simulink library "unifier_obm"  (R2023a)
settings: Solver=VariableStepAuto  StartTime=0.0  StopTime=10.0  RelTol=1e-3
undefined symbols (not defined in the file): b, c, dp_DEP, dp_FUSE_FIN, dp_HTU, dp_VTAIL, dp_VTAIL_INDUCED, dp_WING_root, dp_WING_tip, I, m, S, vtail_nodes, wing_nodes, xyz_cg, xyz_DEP
libraries: sharedutil x7, aerolibtransform2 x4, sharedtransform x2, matrix_library x1, shared6dofsys x1, shared6dof x1, simulink x1
(part 2 of 2)

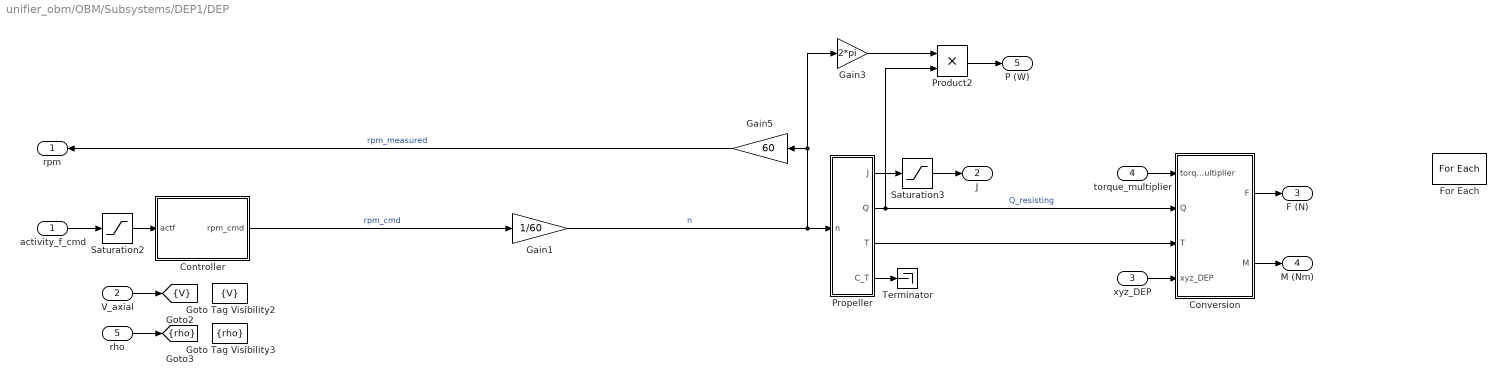
== system unifier_obm/OBM/Subsystems/DEP1/DEP ==
  activity_f_cmd : Inport  Partition=on  PartitionDimension=1  PartitionWidth=1  PartitionOffset=0
  V_axial : Inport  Port=2  Partition=on  PartitionDimension=1  PartitionWidth=1  PartitionOffset=0
  xyz_DEP : Inport  Port=3  Partition=on  PartitionDimension=2  PartitionWidth=1  PartitionOffset=0
  torque_multiplier : Inport  Port=4  Partition=on  PartitionDimension=1  PartitionWidth=1  PartitionOffset=0
  rho : Inport  Port=5
  Controller : Subsystem
  Conversion : Subsystem
  For Each : ForEach  DisableCoverage=on  SpecifiedNumIters=12
  Gain1 : Gain  Gain=1/60
  Gain3 : Gain  Gain=2*pi
  Gain5 : Gain  Gain=60
  Goto Tag Visibility2 : GotoTagVisibility  GotoTag=V
  Goto Tag Visibility3 : GotoTagVisibility  GotoTag=rho
  Product2 : Product
  Propeller : Subsystem
  Saturation2 : Saturate  UpperLimit=1  LowerLimit=0
  Saturation3 : Saturate  UpperLimit=5  LowerLimit=0.2
  Terminator : Terminator
  rpm : Outport  ConcatenationDimension=1
  J : Outport  Port=2  ConcatenationDimension=1
  F (N) : Outport  Port=3  ConcatenationDimension=2
  M (Nm) : Outport  Port=4  ConcatenationDimension=2
  P (W) : Outport  Port=5  ConcatenationDimension=1
  tag scope: V=scoped, rho=scoped
  wires:
  Conversion/1(F) -> F (N)/1
  Conversion/2(M) -> M (Nm)/1
  Saturation3/1 -> J/1
  Propeller/4(C_T) -> Terminator/1
  activity_f_cmd/1 -> Saturation2/1
  Propeller/1(J) -> Saturation3/1
  Gain3/1 -> Product2/1
  xyz_DEP/1 -> Conversion/4(xyz_DEP)
  Gain1/1 -> Gain3/1, Gain5/1, Propeller/1(n)  "n"
  V_axial/1 -> [V]
  Product2/1 -> P (W)/1
  torque_multiplier/1 -> Conversion/1(torque_multiplier)
  Gain5/1 -> rpm/1  "rpm_measured"
  Propeller/3(T) -> Conversion/3(T)
  rho/1 -> [rho]
  Propeller/2(Q) -> Product2/2, Conversion/2(Q)  "Q_resisting"
  Saturation2/1 -> Controller/1(actf)
  Controller/1(rpm_cmd) -> Gain1/1  "rpm_cmd"

== system unifier_obm/OBM/Subsystems/HTU/PropAndMotor ==
  Vrw_mag_eas : Inport
  T_cmd (N) : Inport  Port=2
  1-D Lookup Table : Lookup_n-D  NumberOfTableDimensions=1  BreakpointsForDimension1=dp_HTU.limits.V_low_lim  IndexSearchMethod=Linear search  BeginIndexSearchUsingPreviousIndexResult=on  Table=dp_HTU.limits.T_low_lim  InternalRulePriority=Speed  RndMeth=Simplest
  1-D Lookup Table1 : Lookup_n-D  NumberOfTableDimensions=1  BreakpointsForDimension1=dp_HTU.limits.V_up_lim  IndexSearchMethod=Linear search  BeginIndexSearchUsingPreviousIndexResult=on  Table=dp_HTU.limits.T_up_lim  InternalRulePriority=Speed  RndMeth=Simplest
  P lookup : Lookup_n-D  BreakpointsForDimension1=dp_HTU.V_vec  BreakpointsForDimension2=dp_HTU.T_vec  IndexSearchMethod=Linear search  BeginIndexSearchUsingPreviousIndexResult=on  Table=dp_HTU.P_grid  InternalRulePriority=Speed  RndMeth=Simplest
      settings: InputPortMap=u0,u1
  Saturation Dynamic : simulink/Discontinuities/Saturation Dynamic  OutMin=[]  OutMax=[]  OutDataTypeStr=Inherit: Same as second input  OutDataType=fixdt(1, 16)  OutScaling=2^-10  DoSatur=off
  P (kW) : Outport
  T (N) : Outport  Port=2
  wires:
  Vrw_mag_eas/1 -> P lookup/1, 1-D Lookup Table/1, 1-D Lookup Table1/1
  P lookup/1 -> P (kW)/1
  1-D Lookup Table1/1 -> Saturation Dynamic/1
  1-D Lookup Table/1 -> Saturation Dynamic/3
  T_cmd (N)/1 -> Saturation Dynamic/2
  Saturation Dynamic/1 -> T (N)/1, P lookup/2

== system unifier_obm/OBM/Aero/FinFuselageForces/Subsystem1/Subsystem ==
  beta : Inport
  alpha : Inport  Port=2
  Prelookup : PreLookup  BreakpointsData=dp_FUSE_FIN.beta  IndexSearchMethod=Linear search  BeginIndexSearchUsingPreviousIndexResult=on  ExtrapMethod=Linear
  Prelookup1 : PreLookup  BreakpointsData=dp_FUSE_FIN.aoa  IndexSearchMethod=Linear search  BeginIndexSearchUsingPreviousIndexResult=on  ExtrapMethod=Linear
  Out1 : Outport
  Out2 : Outport  Port=2
  Out3 : Outport  Port=3
  Out4 : Outport  Port=4
  wires:
  Prelookup/1 -> Out1/1
  alpha/1 -> Prelookup1/1
  beta/1 -> Prelookup/1
  Prelookup1/1 -> Out3/1
  Prelookup1/2 -> Out4/1
  Prelookup/2 -> Out2/1

== system unifier_obm/OBM/Aero/VtailForces/Subsystem/CrossProduct1 ==
  r : Inport  Partition=on  PartitionDimension=2  PartitionWidth=1  PartitionOffset=0
  F : Inport  Port=2  Partition=on  PartitionDimension=2  PartitionWidth=1  PartitionOffset=0
  3x3 Cross Product : sharedutil/3x3 Cross Product  aMode=aMode
  CG : Constant  Value=xyz_cg
  Cast : DataTypeConversion  OutDataTypeStr=single  SaturateOnIntegerOverflow=off  RndMeth=Floor
  For Each : ForEach  DisableCoverage=on  SpecifiedNumIters=16
  Minus : Sum  Inputs=+-
  M : Outport  ConcatenationDimension=2
  wires:
  F/1 -> 3x3 Cross Product/2
  r/1 -> Minus/1
  3x3 Cross Product/1 -> M/1
  CG/1 -> Cast/1
  Minus/1 -> 3x3 Cross Product/1
  Cast/1 -> Minus/2

== system unifier_obm/OBM/Aero/VtailForces/VtailForces/WingRootPreLookup ==
  rude_defl_nodes : Inport
  alpha_nodes : Inport  Port=2
  beta_nodes : Inport  Port=3
  Constant8 : Constant  Value=0:15
  Prelookup : PreLookup  BreakpointsData=dp_VTAIL.rude_defl  IndexSearchMethod=Linear search  BeginIndexSearchUsingPreviousIndexResult=on  ExtrapMethod=Linear
  Prelookup1 : PreLookup  BreakpointsData=dp_VTAIL.alphas  IndexSearchMethod=Linear search  BeginIndexSearchUsingPreviousIndexResult=on  ExtrapMethod=Linear
  Prelookup2 : PreLookup  BreakpointsData=dp_VTAIL.betas  IndexSearchMethod=Linear search  BeginIndexSearchUsingPreviousIndexResult=on  ExtrapMethod=Linear
  Out1 : Outport
  Out2 : Outport  Port=2
  Out3 : Outport  Port=3
  Out4 : Outport  Port=4
  Out6 : Outport  Port=5
  Out7 : Outport  Port=6
  Out5 : Outport  Port=7
  wires:
  Prelookup/1 -> Out1/1
  Constant8/1 -> Out5/1
  Prelookup1/2 -> Out4/1
  Prelookup/2 -> Out2/1
  alpha_nodes/1 -> Prelookup1/1
  Prelookup1/1 -> Out3/1
  rude_defl_nodes/1 -> Prelookup/1
  beta_nodes/1 -> Prelookup2/1
  Prelookup2/1 -> Out6/1
  Prelookup2/2 -> Out7/1

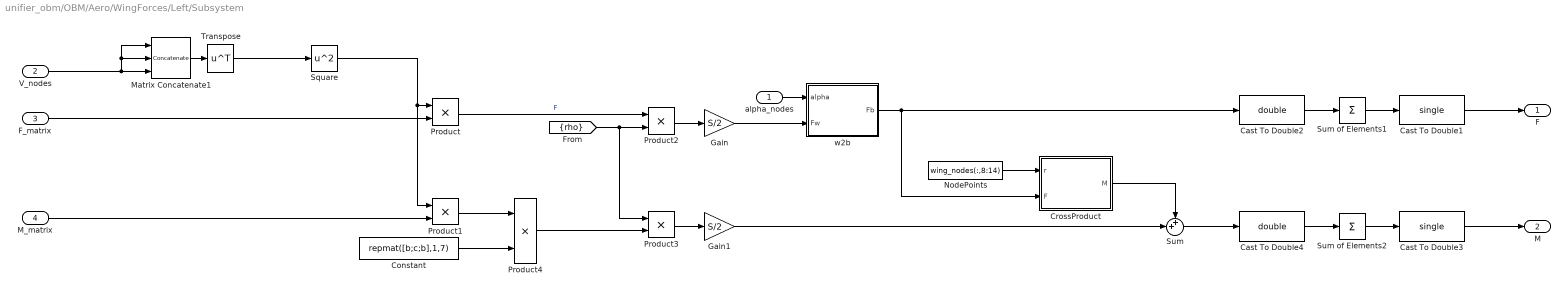
== system unifier_obm/OBM/Aero/WingForces/Left/Subsystem ==
  alpha_nodes : Inport
  V_nodes : Inport  Port=2
  F_matrix : Inport  Port=3
  M_matrix : Inport  Port=4
  Cast To Double1 : DataTypeConversion  OutDataTypeStr=single  SaturateOnIntegerOverflow=off  RndMeth=Floor
  Cast To Double2 : DataTypeConversion  OutDataTypeStr=double  SaturateOnIntegerOverflow=off  RndMeth=Floor
  Cast To Double3 : DataTypeConversion  OutDataTypeStr=single  SaturateOnIntegerOverflow=off  RndMeth=Floor
  Cast To Double4 : DataTypeConversion  OutDataTypeStr=double  SaturateOnIntegerOverflow=off  RndMeth=Floor
  Constant : Constant  Value=repmat([b;c;b],1,7)
  CrossProduct : Subsystem  TreatAsAtomicUnit=on
  Gain : Gain  Gain=S/2
  Gain1 : Gain  Gain=S/2
  Matrix Concatenate1 : Concatenate  NumInputs=3  Mode=Multidimensional array  ConcatenateDimension=2
  NodePoints : Constant  Value=wing_nodes(:,8:14)
  Product{,1..4} (5 alike) : Product
  Square : Math  Operator=square
  Sum : Sum  Inputs=++|
  Sum of Elements1 : Sum  Inputs=+  CollapseMode=Specified dimension  CollapseDim=2
  Sum of Elements2 : Sum  Inputs=+  CollapseMode=Specified dimension  CollapseDim=2
  Transpose : Math  Operator=transpose
  w2b : Subsystem  TreatAsAtomicUnit=on
  F : Outport
  M : Outport  Port=2
  wires:
  Product2/1 -> Gain/1
  F_matrix/1 -> Product/2
  [rho] -> Product3/1, Product2/2
  Product3/1 -> Gain1/1
  Constant/1 -> Product4/2
  Product4/1 -> Product3/2
  M_matrix/1 -> Product1/2
  Product1/1 -> Product4/1
  Gain1/1 -> Sum/2
  Product/1 -> Product2/1  "F"
  V_nodes/1 -> Matrix Concatenate1/1, Matrix Concatenate1/2, Matrix Concatenate1/3
  Transpose/1 -> Square/1
  Matrix Concatenate1/1 -> Transpose/1
  Square/1 -> Product1/1, Product/1
  w2b/1(Fb) -> Cast To Double2/1, CrossProduct/2(F)
  NodePoints/1 -> CrossProduct/1(r)
  CrossProduct/1(M) -> Sum/1
  Cast To Double1/1 -> F/1
  Gain/1 -> w2b/2(Fw)
  alpha_nodes/1 -> w2b/1(alpha)
  Cast To Double2/1 -> Sum of Elements1/1
  Sum of Elements1/1 -> Cast To Double1/1
  Sum of Elements2/1 -> Cast To Double3/1
  Cast To Double4/1 -> Sum of Elements2/1
  Sum/1 -> Cast To Double4/1
  Cast To Double3/1 -> M/1

== system unifier_obm/OBM/Aero/WingForces/Left/WingRootForces ==
  flap_defl : Inport
  alpha : Inport  Port=2
  V_node : Inport  Port=3
  DEP_J : Inport  Port=4
  Interpolation Using Prelookup1 : Interpolation_n-D  NumberOfTableDimensions=5  Table=dp_WING_root.CD  ExtrapMethod=Clip  ValidIndexMayReachLast=on  NumSelectionDims=1  InternalRulePriority=Speed  TableDataTypeStr=Inherit: Inherit from 'Table data'
      settings: InputPortMap=u0,u1,u2,u3,u4,u5,u6,u7,u8
  Interpolation Using Prelookup2 : Interpolation_n-D  NumberOfTableDimensions=5  Table=dp_WING_root.CS  ExtrapMethod=Clip  ValidIndexMayReachLast=on  NumSelectionDims=1  InternalRulePriority=Speed  TableDataTypeStr=Inherit: Inherit from 'Table data'
      settings: InputPortMap=u0,u1,u2,u3,u4,u5,u6,u7,u8
  Interpolation Using Prelookup3 : Interpolation_n-D  NumberOfTableDimensions=5  Table=dp_WING_root.CL  ExtrapMethod=Clip  ValidIndexMayReachLast=on  NumSelectionDims=1  InternalRulePriority=Speed  TableDataTypeStr=Inherit: Inherit from 'Table data'
      settings: InputPortMap=u0,u1,u2,u3,u4,u5,u6,u7,u8
  Interpolation Using Prelookup4 : Interpolation_n-D  NumberOfTableDimensions=5  Table=dp_WING_root.CMx  ExtrapMethod=Clip  ValidIndexMayReachLast=on  NumSelectionDims=1  InternalRulePriority=Speed  TableDataTypeStr=Inherit: Inherit from 'Table data'
      settings: InputPortMap=u0,u1,u2,u3,u4,u5,u6,u7,u8
  Interpolation Using Prelookup5 : Interpolation_n-D  NumberOfTableDimensions=5  Table=dp_WING_root.CMy  ExtrapMethod=Clip  ValidIndexMayReachLast=on  NumSelectionDims=1  InternalRulePriority=Speed  TableDataTypeStr=Inherit: Inherit from 'Table data'
      settings: InputPortMap=u0,u1,u2,u3,u4,u5,u6,u7,u8
  Interpolation Using Prelookup6 : Interpolation_n-D  NumberOfTableDimensions=5  Table=dp_WING_root.CMz  ExtrapMethod=Clip  ValidIndexMayReachLast=on  NumSelectionDims=1  InternalRulePriority=Speed  TableDataTypeStr=Inherit: Inherit from 'Table data'
      settings: InputPortMap=u0,u1,u2,u3,u4,u5,u6,u7,u8
  WingRootPreLookup : Subsystem
  CD : Outport
  CS : Outport  Port=2
  CL : Outport  Port=3
  CMx : Outport  Port=4
  CMy : Outport  Port=5
  CMz : Outport  Port=6
  wires:
  WingRootPreLookup/9(Out5) -> Interpolation Using Prelookup6/9, Interpolation Using Prelookup5/9, Interpolation Using Prelookup4/9, Interpolation Using Prelookup3/9, Interpolation Using Prelookup2/9, Interpolation Using Prelookup1/9
  WingRootPreLookup/3(Out3) -> Interpolation Using Prelookup6/3, Interpolation Using Prelookup5/3, Interpolation Using Prelookup4/3, Interpolation Using Prelookup3/3, Interpolation Using Prelookup2/3, Interpolation Using Prelookup1/3
  WingRootPreLookup/8(Out9) -> Interpolation Using Prelookup6/8, Interpolation Using Prelookup5/8, Interpolation Using Prelookup4/8, Interpolation Using Prelookup3/8, Interpolation Using Prelookup2/8, Interpolation Using Prelookup1/8
  WingRootPreLookup/1(Out1) -> Interpolation Using Prelookup6/1, Interpolation Using Prelookup5/1, Interpolation Using Prelookup4/1, Interpolation Using Prelookup3/1, Interpolation Using Prelookup2/1, Interpolation Using Prelookup1/1
  WingRootPreLookup/7(Out8) -> Interpolation Using Prelookup1/7, Interpolation Using Prelookup5/7, Interpolation Using Prelookup6/7, Interpolation Using Prelookup4/7, Interpolation Using Prelookup3/7, Interpolation Using Prelookup2/7
  flap_defl/1 -> WingRootPreLookup/1(flap_defl)
  WingRootPreLookup/4(Out4) -> Interpolation Using Prelookup6/4, Interpolation Using Prelookup5/4, Interpolation Using Prelookup4/4, Interpolation Using Prelookup3/4, Interpolation Using Prelookup2/4, Interpolation Using Prelookup1/4
  WingRootPreLookup/5(Out6) -> Interpolation Using Prelookup1/5, Interpolation Using Prelookup6/5, Interpolation Using Prelookup5/5, Interpolation Using Prelookup4/5, Interpolation Using Prelookup3/5, Interpolation Using Prelookup2/5
  Interpolation Using Prelookup1/1 -> CD/1
  WingRootPreLookup/6(Out7) -> Interpolation Using Prelookup6/6, Interpolation Using Prelookup5/6, Interpolation Using Prelookup4/6, Interpolation Using Prelookup3/6, Interpolation Using Prelookup2/6, Interpolation Using Prelookup1/6
  WingRootPreLookup/2(Out2) -> Interpolation Using Prelookup6/2, Interpolation Using Prelookup5/2, Interpolation Using Prelookup4/2, Interpolation Using Prelookup3/2, Interpolation Using Prelookup2/2, Interpolation Using Prelookup1/2
  DEP_J/1 -> WingRootPreLookup/4(DEP_J)
  V_node/1 -> WingRootPreLookup/3(V_node)
  alpha/1 -> WingRootPreLookup/2(alpha)
  Interpolation Using Prelookup2/1 -> CS/1
  Interpolation Using Prelookup3/1 -> CL/1
  Interpolation Using Prelookup4/1 -> CMx/1
  Interpolation Using Prelookup5/1 -> CMy/1
  Interpolation Using Prelookup6/1 -> CMz/1

== system unifier_obm/OBM/Aero/WingForces/Left/WingTipForces ==
  ail_defl : Inport
  alpha : Inport  Port=2
  V_node : Inport  Port=3
  DEP_J : Inport  Port=4
  Interpolation Using Prelookup1 : Interpolation_n-D  NumberOfTableDimensions=5  Table=dp_WING_tip.CD  ExtrapMethod=Clip  ValidIndexMayReachLast=on  NumSelectionDims=1  InternalRulePriority=Speed  TableDataTypeStr=Inherit: Inherit from 'Table data'
      settings: InputPortMap=u0,u1,u2,u3,u4,u5,u6,u7,u8
  Interpolation Using Prelookup2 : Interpolation_n-D  NumberOfTableDimensions=5  Table=dp_WING_tip.CS  ExtrapMethod=Clip  ValidIndexMayReachLast=on  NumSelectionDims=1  InternalRulePriority=Speed  TableDataTypeStr=Inherit: Inherit from 'Table data'
      settings: InputPortMap=u0,u1,u2,u3,u4,u5,u6,u7,u8
  Interpolation Using Prelookup3 : Interpolation_n-D  NumberOfTableDimensions=5  Table=dp_WING_tip.CL  ExtrapMethod=Clip  ValidIndexMayReachLast=on  NumSelectionDims=1  InternalRulePriority=Speed  TableDataTypeStr=Inherit: Inherit from 'Table data'
      settings: InputPortMap=u0,u1,u2,u3,u4,u5,u6,u7,u8
  Interpolation Using Prelookup4 : Interpolation_n-D  NumberOfTableDimensions=5  Table=dp_WING_tip.CMx  ExtrapMethod=Clip  ValidIndexMayReachLast=on  NumSelectionDims=1  InternalRulePriority=Speed  TableDataTypeStr=Inherit: Inherit from 'Table data'
      settings: InputPortMap=u0,u1,u2,u3,u4,u5,u6,u7,u8
  Interpolation Using Prelookup5 : Interpolation_n-D  NumberOfTableDimensions=5  Table=dp_WING_tip.CMy  ExtrapMethod=Clip  ValidIndexMayReachLast=on  NumSelectionDims=1  InternalRulePriority=Speed  TableDataTypeStr=Inherit: Inherit from 'Table data'
      settings: InputPortMap=u0,u1,u2,u3,u4,u5,u6,u7,u8
  Interpolation Using Prelookup6 : Interpolation_n-D  NumberOfTableDimensions=5  Table=dp_WING_tip.CMz  ExtrapMethod=Clip  ValidIndexMayReachLast=on  NumSelectionDims=1  InternalRulePriority=Speed  TableDataTypeStr=Inherit: Inherit from 'Table data'
      settings: InputPortMap=u0,u1,u2,u3,u4,u5,u6,u7,u8
  WingRootPreLookup : Subsystem
  CD : Outport
  CS : Outport  Port=2
  CL : Outport  Port=3
  CMx : Outport  Port=4
  CMy : Outport  Port=5
  CMz : Outport  Port=6
  wires:
  WingRootPreLookup/9(Out5) -> Interpolation Using Prelookup6/9, Interpolation Using Prelookup5/9, Interpolation Using Prelookup4/9, Interpolation Using Prelookup3/9, Interpolation Using Prelookup2/9, Interpolation Using Prelookup1/9
  WingRootPreLookup/3(Out3) -> Interpolation Using Prelookup6/3, Interpolation Using Prelookup5/3, Interpolation Using Prelookup4/3, Interpolation Using Prelookup3/3, Interpolation Using Prelookup2/3, Interpolation Using Prelookup1/3
  WingRootPreLookup/8(Out9) -> Interpolation Using Prelookup6/8, Interpolation Using Prelookup5/8, Interpolation Using Prelookup4/8, Interpolation Using Prelookup3/8, Interpolation Using Prelookup2/8, Interpolation Using Prelookup1/8
  WingRootPreLookup/1(Out1) -> Interpolation Using Prelookup6/1, Interpolation Using Prelookup5/1, Interpolation Using Prelookup4/1, Interpolation Using Prelookup3/1, Interpolation Using Prelookup2/1, Interpolation Using Prelookup1/1
  WingRootPreLookup/7(Out8) -> Interpolation Using Prelookup5/7, Interpolation Using Prelookup6/7, Interpolation Using Prelookup4/7, Interpolation Using Prelookup3/7, Interpolation Using Prelookup2/7, Interpolation Using Prelookup1/7
  ail_defl/1 -> WingRootPreLookup/1(ail_defl)
  WingRootPreLookup/4(Out4) -> Interpolation Using Prelookup6/4, Interpolation Using Prelookup5/4, Interpolation Using Prelookup4/4, Interpolation Using Prelookup3/4, Interpolation Using Prelookup2/4, Interpolation Using Prelookup1/4
  WingRootPreLookup/5(Out6) -> Interpolation Using Prelookup1/5, Interpolation Using Prelookup6/5, Interpolation Using Prelookup5/5, Interpolation Using Prelookup4/5, Interpolation Using Prelookup3/5, Interpolation Using Prelookup2/5
  Interpolation Using Prelookup1/1 -> CD/1
  WingRootPreLookup/6(Out7) -> Interpolation Using Prelookup6/6, Interpolation Using Prelookup5/6, Interpolation Using Prelookup4/6, Interpolation Using Prelookup3/6, Interpolation Using Prelookup2/6, Interpolation Using Prelookup1/6
  WingRootPreLookup/2(Out2) -> Interpolation Using Prelookup6/2, Interpolation Using Prelookup5/2, Interpolation Using Prelookup4/2, Interpolation Using Prelookup3/2, Interpolation Using Prelookup2/2, Interpolation Using Prelookup1/2
  DEP_J/1 -> WingRootPreLookup/4(DEP_J)
  V_node/1 -> WingRootPreLookup/3(V_node)
  alpha/1 -> WingRootPreLookup/2(alpha)
  Interpolation Using Prelookup2/1 -> CS/1
  Interpolation Using Prelookup3/1 -> CL/1
  Interpolation Using Prelookup4/1 -> CMx/1
  Interpolation Using Prelookup5/1 -> CMy/1
  Interpolation Using Prelookup6/1 -> CMz/1

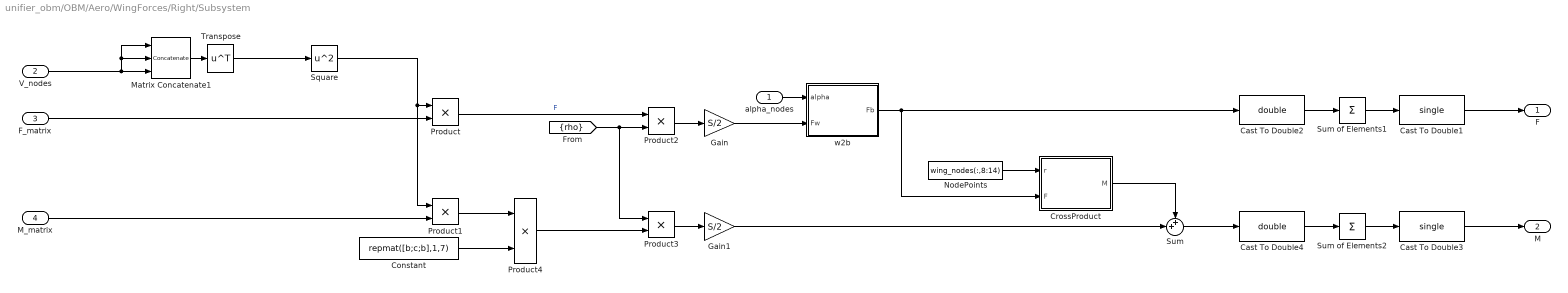
== system unifier_obm/OBM/Aero/WingForces/Right/Subsystem ==
  alpha_nodes : Inport
  V_nodes : Inport  Port=2
  F_matrix : Inport  Port=3
  M_matrix : Inport  Port=4
  Cast To Double1 : DataTypeConversion  OutDataTypeStr=single  SaturateOnIntegerOverflow=off  RndMeth=Floor
  Cast To Double2 : DataTypeConversion  OutDataTypeStr=double  SaturateOnIntegerOverflow=off  RndMeth=Floor
  Cast To Double3 : DataTypeConversion  OutDataTypeStr=single  SaturateOnIntegerOverflow=off  RndMeth=Floor
  Cast To Double4 : DataTypeConversion  OutDataTypeStr=double  SaturateOnIntegerOverflow=off  RndMeth=Floor
  Constant : Constant  Value=repmat([b;c;b],1,7)
  CrossProduct : Subsystem  TreatAsAtomicUnit=on
  Gain : Gain  Gain=S/2
  Gain1 : Gain  Gain=S/2
  Matrix Concatenate1 : Concatenate  NumInputs=3  Mode=Multidimensional array  ConcatenateDimension=2
  NodePoints : Constant  Value=wing_nodes(:,8:14)
  Product{,1..4} (5 alike) : Product
  Square : Math  Operator=square
  Sum : Sum  Inputs=++|
  Sum of Elements1 : Sum  Inputs=+  CollapseMode=Specified dimension  CollapseDim=2
  Sum of Elements2 : Sum  Inputs=+  CollapseMode=Specified dimension  CollapseDim=2
  Transpose : Math  Operator=transpose
  w2b : Subsystem  TreatAsAtomicUnit=on
  F : Outport
  M : Outport  Port=2
  wires:
  Product2/1 -> Gain/1
  F_matrix/1 -> Product/2
  [rho] -> Product3/1, Product2/2
  Product3/1 -> Gain1/1
  Constant/1 -> Product4/2
  Product4/1 -> Product3/2
  M_matrix/1 -> Product1/2
  Product1/1 -> Product4/1
  Gain1/1 -> Sum/2
  Product/1 -> Product2/1  "F"
  V_nodes/1 -> Matrix Concatenate1/1, Matrix Concatenate1/2, Matrix Concatenate1/3
  Transpose/1 -> Square/1
  Matrix Concatenate1/1 -> Transpose/1
  Square/1 -> Product1/1, Product/1
  w2b/1(Fb) -> Cast To Double2/1, CrossProduct/2(F)
  NodePoints/1 -> CrossProduct/1(r)
  CrossProduct/1(M) -> Sum/1
  Cast To Double1/1 -> F/1
  Gain/1 -> w2b/2(Fw)
  alpha_nodes/1 -> w2b/1(alpha)
  Cast To Double2/1 -> Sum of Elements1/1
  Sum of Elements1/1 -> Cast To Double1/1
  Sum of Elements2/1 -> Cast To Double3/1
  Cast To Double4/1 -> Sum of Elements2/1
  Sum/1 -> Cast To Double4/1
  Cast To Double3/1 -> M/1

== system unifier_obm/OBM/Aero/WingForces/Right/WingRootForces ==
  flap_defl : Inport
  alpha : Inport  Port=2
  V_node : Inport  Port=3
  DEP_J : Inport  Port=4
  Interpolation Using Prelookup1 : Interpolation_n-D  NumberOfTableDimensions=5  Table=dp_WING_root.CD  ExtrapMethod=Clip  ValidIndexMayReachLast=on  NumSelectionDims=1  InternalRulePriority=Speed  TableDataTypeStr=Inherit: Inherit from 'Table data'
      settings: InputPortMap=u0,u1,u2,u3,u4,u5,u6,u7,u8
  Interpolation Using Prelookup2 : Interpolation_n-D  NumberOfTableDimensions=5  Table=dp_WING_root.CS  ExtrapMethod=Clip  ValidIndexMayReachLast=on  NumSelectionDims=1  InternalRulePriority=Speed  TableDataTypeStr=Inherit: Inherit from 'Table data'
      settings: InputPortMap=u0,u1,u2,u3,u4,u5,u6,u7,u8
  Interpolation Using Prelookup3 : Interpolation_n-D  NumberOfTableDimensions=5  Table=dp_WING_root.CL  ExtrapMethod=Clip  ValidIndexMayReachLast=on  NumSelectionDims=1  InternalRulePriority=Speed  TableDataTypeStr=Inherit: Inherit from 'Table data'
      settings: InputPortMap=u0,u1,u2,u3,u4,u5,u6,u7,u8
  Interpolation Using Prelookup4 : Interpolation_n-D  NumberOfTableDimensions=5  Table=dp_WING_root.CMx  ExtrapMethod=Clip  ValidIndexMayReachLast=on  NumSelectionDims=1  InternalRulePriority=Speed  TableDataTypeStr=Inherit: Inherit from 'Table data'
      settings: InputPortMap=u0,u1,u2,u3,u4,u5,u6,u7,u8
  Interpolation Using Prelookup5 : Interpolation_n-D  NumberOfTableDimensions=5  Table=dp_WING_root.CMy  ExtrapMethod=Clip  ValidIndexMayReachLast=on  NumSelectionDims=1  InternalRulePriority=Speed  TableDataTypeStr=Inherit: Inherit from 'Table data'
      settings: InputPortMap=u0,u1,u2,u3,u4,u5,u6,u7,u8
  Interpolation Using Prelookup6 : Interpolation_n-D  NumberOfTableDimensions=5  Table=dp_WING_root.CMz  ExtrapMethod=Clip  ValidIndexMayReachLast=on  NumSelectionDims=1  InternalRulePriority=Speed  TableDataTypeStr=Inherit: Inherit from 'Table data'
      settings: InputPortMap=u0,u1,u2,u3,u4,u5,u6,u7,u8
  WingRootPreLookup : Subsystem
  CD : Outport
  CS : Outport  Port=2
  CL : Outport  Port=3
  CMx : Outport  Port=4
  CMy : Outport  Port=5
  CMz : Outport  Port=6
  wires:
  WingRootPreLookup/9(Out5) -> Interpolation Using Prelookup6/9, Interpolation Using Prelookup5/9, Interpolation Using Prelookup4/9, Interpolation Using Prelookup3/9, Interpolation Using Prelookup2/9, Interpolation Using Prelookup1/9
  WingRootPreLookup/3(Out3) -> Interpolation Using Prelookup6/3, Interpolation Using Prelookup5/3, Interpolation Using Prelookup4/3, Interpolation Using Prelookup3/3, Interpolation Using Prelookup2/3, Interpolation Using Prelookup1/3
  WingRootPreLookup/8(Out9) -> Interpolation Using Prelookup6/8, Interpolation Using Prelookup5/8, Interpolation Using Prelookup4/8, Interpolation Using Prelookup3/8, Interpolation Using Prelookup2/8, Interpolation Using Prelookup1/8
  WingRootPreLookup/1(Out1) -> Interpolation Using Prelookup6/1, Interpolation Using Prelookup5/1, Interpolation Using Prelookup4/1, Interpolation Using Prelookup3/1, Interpolation Using Prelookup2/1, Interpolation Using Prelookup1/1
  WingRootPreLookup/7(Out8) -> Interpolation Using Prelookup1/7, Interpolation Using Prelookup5/7, Interpolation Using Prelookup6/7, Interpolation Using Prelookup4/7, Interpolation Using Prelookup3/7, Interpolation Using Prelookup2/7
  flap_defl/1 -> WingRootPreLookup/1(flap_defl)
  WingRootPreLookup/4(Out4) -> Interpolation Using Prelookup6/4, Interpolation Using Prelookup5/4, Interpolation Using Prelookup4/4, Interpolation Using Prelookup3/4, Interpolation Using Prelookup2/4, Interpolation Using Prelookup1/4
  WingRootPreLookup/5(Out6) -> Interpolation Using Prelookup1/5, Interpolation Using Prelookup6/5, Interpolation Using Prelookup5/5, Interpolation Using Prelookup4/5, Interpolation Using Prelookup3/5, Interpolation Using Prelookup2/5
  Interpolation Using Prelookup1/1 -> CD/1
  WingRootPreLookup/6(Out7) -> Interpolation Using Prelookup6/6, Interpolation Using Prelookup5/6, Interpolation Using Prelookup4/6, Interpolation Using Prelookup3/6, Interpolation Using Prelookup2/6, Interpolation Using Prelookup1/6
  WingRootPreLookup/2(Out2) -> Interpolation Using Prelookup6/2, Interpolation Using Prelookup5/2, Interpolation Using Prelookup4/2, Interpolation Using Prelookup3/2, Interpolation Using Prelookup2/2, Interpolation Using Prelookup1/2
  DEP_J/1 -> WingRootPreLookup/4(DEP_J)
  V_node/1 -> WingRootPreLookup/3(V_node)
  alpha/1 -> WingRootPreLookup/2(alpha)
  Interpolation Using Prelookup2/1 -> CS/1
  Interpolation Using Prelookup3/1 -> CL/1
  Interpolation Using Prelookup4/1 -> CMx/1
  Interpolation Using Prelookup5/1 -> CMy/1
  Interpolation Using Prelookup6/1 -> CMz/1

== system unifier_obm/OBM/Aero/WingForces/Right/WingTipForces ==
  ail_defl : Inport
  alpha : Inport  Port=2
  V_node : Inport  Port=3
  DEP_J : Inport  Port=4
  Interpolation Using Prelookup1 : Interpolation_n-D  NumberOfTableDimensions=5  Table=dp_WING_tip.CD  ExtrapMethod=Clip  ValidIndexMayReachLast=on  NumSelectionDims=1  InternalRulePriority=Speed  TableDataTypeStr=Inherit: Inherit from 'Table data'
      settings: InputPortMap=u0,u1,u2,u3,u4,u5,u6,u7,u8
  Interpolation Using Prelookup2 : Interpolation_n-D  NumberOfTableDimensions=5  Table=dp_WING_tip.CS  ExtrapMethod=Clip  ValidIndexMayReachLast=on  NumSelectionDims=1  InternalRulePriority=Speed  TableDataTypeStr=Inherit: Inherit from 'Table data'
      settings: InputPortMap=u0,u1,u2,u3,u4,u5,u6,u7,u8
  Interpolation Using Prelookup3 : Interpolation_n-D  NumberOfTableDimensions=5  Table=dp_WING_tip.CL  ExtrapMethod=Clip  ValidIndexMayReachLast=on  NumSelectionDims=1  InternalRulePriority=Speed  TableDataTypeStr=Inherit: Inherit from 'Table data'
      settings: InputPortMap=u0,u1,u2,u3,u4,u5,u6,u7,u8
  Interpolation Using Prelookup4 : Interpolation_n-D  NumberOfTableDimensions=5  Table=dp_WING_tip.CMx  ExtrapMethod=Clip  ValidIndexMayReachLast=on  NumSelectionDims=1  InternalRulePriority=Speed  TableDataTypeStr=Inherit: Inherit from 'Table data'
      settings: InputPortMap=u0,u1,u2,u3,u4,u5,u6,u7,u8
  Interpolation Using Prelookup5 : Interpolation_n-D  NumberOfTableDimensions=5  Table=dp_WING_tip.CMy  ExtrapMethod=Clip  ValidIndexMayReachLast=on  NumSelectionDims=1  InternalRulePriority=Speed  TableDataTypeStr=Inherit: Inherit from 'Table data'
      settings: InputPortMap=u0,u1,u2,u3,u4,u5,u6,u7,u8
  Interpolation Using Prelookup6 : Interpolation_n-D  NumberOfTableDimensions=5  Table=dp_WING_tip.CMz  ExtrapMethod=Clip  ValidIndexMayReachLast=on  NumSelectionDims=1  InternalRulePriority=Speed  TableDataTypeStr=Inherit: Inherit from 'Table data'
      settings: InputPortMap=u0,u1,u2,u3,u4,u5,u6,u7,u8
  WingRootPreLookup : Subsystem
  CD : Outport
  CS : Outport  Port=2
  CL : Outport  Port=3
  CMx : Outport  Port=4
  CMy : Outport  Port=5
  CMz : Outport  Port=6
  wires:
  WingRootPreLookup/9(Out5) -> Interpolation Using Prelookup6/9, Interpolation Using Prelookup5/9, Interpolation Using Prelookup4/9, Interpolation Using Prelookup3/9, Interpolation Using Prelookup2/9, Interpolation Using Prelookup1/9
  WingRootPreLookup/3(Out3) -> Interpolation Using Prelookup6/3, Interpolation Using Prelookup5/3, Interpolation Using Prelookup4/3, Interpolation Using Prelookup3/3, Interpolation Using Prelookup2/3, Interpolation Using Prelookup1/3
  WingRootPreLookup/8(Out9) -> Interpolation Using Prelookup6/8, Interpolation Using Prelookup5/8, Interpolation Using Prelookup4/8, Interpolation Using Prelookup3/8, Interpolation Using Prelookup2/8, Interpolation Using Prelookup1/8
  WingRootPreLookup/1(Out1) -> Interpolation Using Prelookup6/1, Interpolation Using Prelookup5/1, Interpolation Using Prelookup4/1, Interpolation Using Prelookup3/1, Interpolation Using Prelookup2/1, Interpolation Using Prelookup1/1
  WingRootPreLookup/7(Out8) -> Interpolation Using Prelookup5/7, Interpolation Using Prelookup6/7, Interpolation Using Prelookup4/7, Interpolation Using Prelookup3/7, Interpolation Using Prelookup2/7, Interpolation Using Prelookup1/7
  ail_defl/1 -> WingRootPreLookup/1(ail_defl)
  WingRootPreLookup/4(Out4) -> Interpolation Using Prelookup6/4, Interpolation Using Prelookup5/4, Interpolation Using Prelookup4/4, Interpolation Using Prelookup3/4, Interpolation Using Prelookup2/4, Interpolation Using Prelookup1/4
  WingRootPreLookup/5(Out6) -> Interpolation Using Prelookup1/5, Interpolation Using Prelookup6/5, Interpolation Using Prelookup5/5, Interpolation Using Prelookup4/5, Interpolation Using Prelookup3/5, Interpolation Using Prelookup2/5
  Interpolation Using Prelookup1/1 -> CD/1
  WingRootPreLookup/6(Out7) -> Interpolation Using Prelookup6/6, Interpolation Using Prelookup5/6, Interpolation Using Prelookup4/6, Interpolation Using Prelookup3/6, Interpolation Using Prelookup2/6, Interpolation Using Prelookup1/6
  WingRootPreLookup/2(Out2) -> Interpolation Using Prelookup6/2, Interpolation Using Prelookup5/2, Interpolation Using Prelookup4/2, Interpolation Using Prelookup3/2, Interpolation Using Prelookup2/2, Interpolation Using Prelookup1/2
  DEP_J/1 -> WingRootPreLookup/4(DEP_J)
  V_node/1 -> WingRootPreLookup/3(V_node)
  alpha/1 -> WingRootPreLookup/2(alpha)
  Interpolation Using Prelookup2/1 -> CS/1
  Interpolation Using Prelookup3/1 -> CL/1
  Interpolation Using Prelookup4/1 -> CMx/1
  Interpolation Using Prelookup5/1 -> CMy/1
  Interpolation Using Prelookup6/1 -> CMz/1

== system unifier_obm/OBM/Subsystems/DEP1/DEP/Controller ==
  actf : Inport
  Constant3 : Constant  Value=0
  Switch1 : Switch  Criteria=u2 > Threshold  Threshold=0.001  SaturateOnIntegerOverflow=off  InputSameDT=off
  T2rpm : Lookup_n-D  BreakpointsForDimension1=dp_DEP.rpm_lookup.V_vec  BreakpointsForDimension2=dp_DEP.rpm_lookup.T_vec  IndexSearchMethod=Linear search  BeginIndexSearchUsingPreviousIndexResult=on  Table=dp_DEP.rpm_lookup.rpm_gird  ExtrapMethod=Clip  InternalRulePriority=Speed  RndMeth=Simplest
      settings: InputPortMap=u0,u1
  actf2T : Gain  Gain=800
  rpm_cmd : Outport
  wires:
  actf2T/1 -> T2rpm/2
  Constant3/1 -> Switch1/3
  Switch1/1 -> rpm_cmd/1
  actf/1 -> Switch1/2, actf2T/1
  [V] -> T2rpm/1
  T2rpm/1 -> Switch1/1

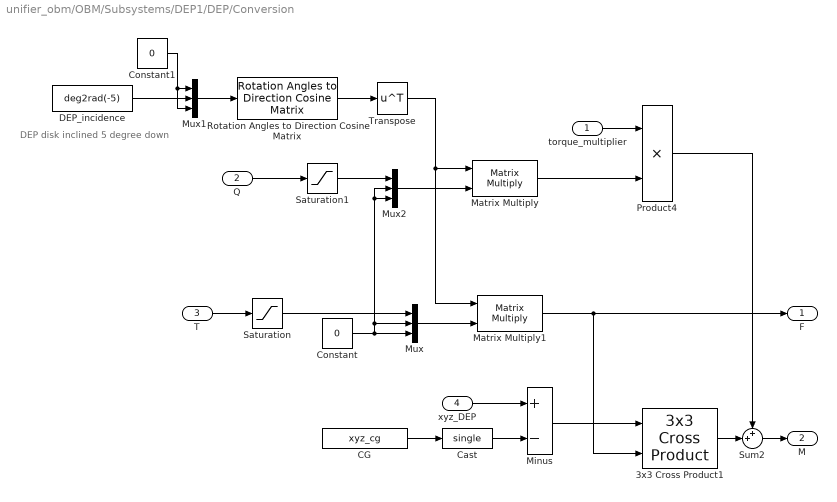
== system unifier_obm/OBM/Subsystems/DEP1/DEP/Conversion ==
  note: DEP disk inclined 5 degree down
  torque_multiplier : Inport
  Q : Inport  Port=2
  T : Inport  Port=3
  xyz_DEP : Inport  Port=4
  3x3 Cross Product1 : sharedutil/3x3 Cross Product  aMode=aMode
  CG : Constant  Value=xyz_cg
  Cast : DataTypeConversion  OutDataTypeStr=single  SaturateOnIntegerOverflow=off  RndMeth=Floor
  Constant : Constant  Value=0
  Constant1 : Constant  Value=0
  DEP_incidence : Constant  Value=deg2rad(-5)
  Matrix Multiply : Product  Multiplication=Matrix(*)
  Matrix Multiply1 : Product  Multiplication=Matrix(*)
  Minus : Sum  Inputs=+-
  Mux : Mux  Inputs=3
  Mux1 : Mux  Inputs=3
  Mux2 : Mux  Inputs=3
  Product4 : Product
  Rotation Angles to Direction Cosine Matrix : sharedtransform/Rotation Angles to Direction Cosine Matrix  rotationOrder=ZYX  aMode=aMode
  Saturation : Saturate  UpperLimit=inf  LowerLimit=0
  Saturation1 : Saturate  UpperLimit=inf  LowerLimit=0
  Sum2 : Sum  Inputs=++|
  Transpose : Math  Operator=transpose
  F : Outport
  M : Outport  Port=2
  wires:
  Rotation Angles to Direction Cosine Matrix/1 -> Transpose/1
  Matrix Multiply/1 -> Product4/2
  Product4/1 -> Sum2/1
  Matrix Multiply1/1 -> F/1, 3x3 Cross Product1/2
  Mux2/1 -> Matrix Multiply/2
  torque_multiplier/1 -> Product4/1
  DEP_incidence/1 -> Mux1/2
  Cast/1 -> Minus/2
  Constant1/1 -> Mux1/3, Mux1/1
  Minus/1 -> 3x3 Cross Product1/1
  Mux1/1 -> Rotation Angles to Direction Cosine Matrix/1
  Mux/1 -> Matrix Multiply1/2
  xyz_DEP/1 -> Minus/1
  CG/1 -> Cast/1
  3x3 Cross Product1/1 -> Sum2/2
  Saturation/1 -> Mux/1
  Sum2/1 -> M/1
  Constant/1 -> Mux/3, Mux2/3, Mux2/2, Mux/2
  Q/1 -> Saturation1/1
  Transpose/1 -> Matrix Multiply1/1, Matrix Multiply/1
  T/1 -> Saturation/1
  Saturation1/1 -> Mux2/1

== system unifier_obm/OBM/Subsystems/DEP1/DEP/Propeller ==
  n : Inport
  Constant : Constant  Value=eps
  Divide : Product  Inputs=*/
  Gain : Gain  Gain=1.6^5
  Gain2 : Gain  Gain=1.6
  Gain3 : Gain  Gain=1.6^4
  Product{,1..3} (4 alike) : Product
  Propeller data LOOKUP C_Q : Lookup_n-D  NumberOfTableDimensions=1  BreakpointsForDimension1=dp_DEP.J  IndexSearchMethod=Linear search  BeginIndexSearchUsingPreviousIndexResult=on  Table=dp_DEP.C_Q  ExtrapMethod=Clip  UseLastTableValue=on  InternalRulePriority=Speed  RndMeth=Simplest
  Propeller data LOOKUP C_T : Lookup_n-D  NumberOfTableDimensions=1  BreakpointsForDimension1=dp_DEP.J  IndexSearchMethod=Linear search  BeginIndexSearchUsingPreviousIndexResult=on  Table=dp_DEP.C_T  ExtrapMethod=Clip  UseLastTableValue=on  InternalRulePriority=Speed  RndMeth=Simplest
  Saturation : Saturate  UpperLimit=inf  LowerLimit=0
  Saturation1 : Saturate  UpperLimit=2.5  LowerLimit=0.3
  Square : Math  Operator=square
  Sum2 : Sum  Inputs=|++
  J : Outport
  Q : Outport  Port=2
  T : Outport  Port=3
  C_T : Outport  Port=4
  wires:
  Product2/1 -> Product3/1
  Sum2/1 -> Divide/2
  [rho] -> Product2/1, Product/1
  Saturation/1 -> Square/1, Gain2/1
  Gain/1 -> Q/1
  Gain3/1 -> T/1
  Divide/1 -> Saturation1/1  "J"
  [V] -> Divide/1
  Constant/1 -> Sum2/2
  Product3/1 -> Gain3/1
  Product1/1 -> Gain/1
  Propeller data LOOKUP C_Q/1 -> Product/2  "C_Q"
  Propeller data LOOKUP C_T/1 -> C_T/1, Product2/2  "C_T"
  Square/1 -> Product3/2, Product1/1
  Product/1 -> Product1/2
  Gain2/1 -> Sum2/1
  Saturation1/1 -> J/1, Propeller data LOOKUP C_Q/1, Propeller data LOOKUP C_T/1
  n/1 -> Saturation/1

== system unifier_obm/OBM/Aero/WingForces/Left/Subsystem/CrossProduct ==
  r : Inport  Partition=on  PartitionDimension=2  PartitionWidth=1  PartitionOffset=0
  F : Inport  Port=2  Partition=on  PartitionDimension=2  PartitionWidth=1  PartitionOffset=0
  3x3 Cross Product : sharedutil/3x3 Cross Product  aMode=aMode
  CG : Constant  Value=xyz_cg
  Cast : DataTypeConversion  OutDataTypeStr=single  SaturateOnIntegerOverflow=off  RndMeth=Floor
  For Each : ForEach  DisableCoverage=on  SpecifiedNumIters=7
  Minus : Sum  Inputs=+-
  M : Outport  ConcatenationDimension=2
  wires:
  F/1 -> 3x3 Cross Product/2
  r/1 -> Minus/1
  3x3 Cross Product/1 -> M/1
  CG/1 -> Cast/1
  Minus/1 -> 3x3 Cross Product/1
  Cast/1 -> Minus/2

== system unifier_obm/OBM/Aero/WingForces/Left/Subsystem/w2b ==
  alpha : Inport  OutDataTypeStr=single  Partition=on  PartitionDimension=1  PartitionWidth=1  PartitionOffset=0
  Fw : Inport  Port=2  Partition=on  PartitionDimension=2  PartitionWidth=1  PartitionOffset=0
  Cast To Double : DataTypeConversion  OutDataTypeStr=double  SaturateOnIntegerOverflow=off  RndMeth=Floor
  Cast To Single : DataTypeConversion  OutDataTypeStr=single  SaturateOnIntegerOverflow=off  RndMeth=Floor
  Constant : Constant  Value=0  OutDataTypeStr=single
  Demux : Demux  Outputs=3
  Direction Cosine Matrix Body to Wind : aerolibtransform2/Direction Cosine Matrix Body to Wind
  For Each : ForEach  DisableCoverage=on  SpecifiedNumIters=7
  Matrix Multiply : Product  Multiplication=Matrix(*)
  Mux : Mux  Inputs=3
  Mux1 : Mux  Inputs=2
  Transpose : Math  Operator=transpose
  Unary Minus : UnaryMinus
  Unary Minus1 : UnaryMinus
  Fb : Outport  ConcatenationDimension=2
  wires:
  Fw/1 -> Demux/1
  alpha/1 -> Mux1/1
  Matrix Multiply/1 -> Fb/1
  Mux/1 -> Matrix Multiply/2
  Demux/1 -> Unary Minus/1
  Unary Minus/1 -> Mux/1
  Demux/2 -> Mux/2
  Unary Minus1/1 -> Mux/3
  Demux/3 -> Unary Minus1/1
  Direction Cosine Matrix Body to Wind/1 -> Transpose/1
  Transpose/1 -> Cast To Single/1
  Mux1/1 -> Cast To Double/1
  Constant/1 -> Mux1/2
  Cast To Single/1 -> Matrix Multiply/1
  Cast To Double/1 -> Direction Cosine Matrix Body to Wind/1

== system unifier_obm/OBM/Aero/WingForces/Left/WingRootForces/WingRootPreLookup ==
  flap_defl : Inport
  alpha : Inport  Port=2
  V_node : Inport  Port=3
  DEP_J : Inport  Port=4
  Constant8 : Constant  Value=0:4
  Prelookup : PreLookup  BreakpointsData=dp_WING_root.flap_defl  IndexSearchMethod=Linear search  BeginIndexSearchUsingPreviousIndexResult=on  UseLastBreakpoint=on
  Prelookup1 : PreLookup  BreakpointsData=dp_WING_root.alphas  IndexSearchMethod=Linear search  BeginIndexSearchUsingPreviousIndexResult=on  UseLastBreakpoint=on
  Prelookup2 : PreLookup  BreakpointsData=dp_WING_root.V  IndexSearchMethod=Linear search  BeginIndexSearchUsingPreviousIndexResult=on  UseLastBreakpoint=on
  Prelookup3 : PreLookup  BreakpointsData=dp_WING_root.DEP_J  IndexSearchMethod=Linear search  BeginIndexSearchUsingPreviousIndexResult=on  UseLastBreakpoint=on
  Out1 : Outport
  Out2 : Outport  Port=2
  Out3 : Outport  Port=3
  Out4 : Outport  Port=4
  Out6 : Outport  Port=5
  Out7 : Outport  Port=6
  Out8 : Outport  Port=7
  Out9 : Outport  Port=8
  Out5 : Outport  Port=9
  wires:
  Prelookup/1 -> Out1/1
  Constant8/1 -> Out5/1
  Prelookup1/2 -> Out4/1
  Prelookup/2 -> Out2/1
  alpha/1 -> Prelookup1/1
  Prelookup1/1 -> Out3/1
  flap_defl/1 -> Prelookup/1
  V_node/1 -> Prelookup2/1
  DEP_J/1 -> Prelookup3/1
  Prelookup2/1 -> Out6/1
  Prelookup2/2 -> Out7/1
  Prelookup3/1 -> Out8/1
  Prelookup3/2 -> Out9/1

== system unifier_obm/OBM/Aero/WingForces/Left/WingTipForces/WingRootPreLookup ==
  ail_defl : Inport
  alpha : Inport  Port=2
  V_node : Inport  Port=3
  DEP_J : Inport  Port=4
  Constant8 : Constant  Value=0:1
  Prelookup : PreLookup  BreakpointsData=dp_WING_tip.ail_defl  IndexSearchMethod=Linear search  BeginIndexSearchUsingPreviousIndexResult=on  UseLastBreakpoint=on
  Prelookup1 : PreLookup  BreakpointsData=dp_WING_tip.alphas  IndexSearchMethod=Linear search  BeginIndexSearchUsingPreviousIndexResult=on  UseLastBreakpoint=on
  Prelookup2 : PreLookup  BreakpointsData=dp_WING_tip.V  IndexSearchMethod=Linear search  BeginIndexSearchUsingPreviousIndexResult=on  UseLastBreakpoint=on
  Prelookup3 : PreLookup  BreakpointsData=dp_WING_tip.DEP_J  IndexSearchMethod=Linear search  BeginIndexSearchUsingPreviousIndexResult=on  UseLastBreakpoint=on
  Out1 : Outport
  Out2 : Outport  Port=2
  Out3 : Outport  Port=3
  Out4 : Outport  Port=4
  Out6 : Outport  Port=5
  Out7 : Outport  Port=6
  Out8 : Outport  Port=7
  Out9 : Outport  Port=8
  Out5 : Outport  Port=9
  wires:
  Prelookup/1 -> Out1/1
  Constant8/1 -> Out5/1
  Prelookup1/2 -> Out4/1
  Prelookup/2 -> Out2/1
  alpha/1 -> Prelookup1/1
  Prelookup1/1 -> Out3/1
  ail_defl/1 -> Prelookup/1
  V_node/1 -> Prelookup2/1
  DEP_J/1 -> Prelookup3/1
  Prelookup2/1 -> Out6/1
  Prelookup2/2 -> Out7/1
  Prelookup3/1 -> Out8/1
  Prelookup3/2 -> Out9/1

== system unifier_obm/OBM/Aero/WingForces/Right/Subsystem/CrossProduct ==
  r : Inport  Partition=on  PartitionDimension=2  PartitionWidth=1  PartitionOffset=0
  F : Inport  Port=2  Partition=on  PartitionDimension=2  PartitionWidth=1  PartitionOffset=0
  3x3 Cross Product : sharedutil/3x3 Cross Product  aMode=aMode
  CG : Constant  Value=xyz_cg
  Cast : DataTypeConversion  OutDataTypeStr=single  SaturateOnIntegerOverflow=off  RndMeth=Floor
  For Each : ForEach  DisableCoverage=on  SpecifiedNumIters=7
  Minus : Sum  Inputs=+-
  M : Outport  ConcatenationDimension=2
  wires:
  F/1 -> 3x3 Cross Product/2
  r/1 -> Minus/1
  3x3 Cross Product/1 -> M/1
  CG/1 -> Cast/1
  Minus/1 -> 3x3 Cross Product/1
  Cast/1 -> Minus/2

== system unifier_obm/OBM/Aero/WingForces/Right/Subsystem/w2b ==
  alpha : Inport  OutDataTypeStr=single  Partition=on  PartitionDimension=1  PartitionWidth=1  PartitionOffset=0
  Fw : Inport  Port=2  Partition=on  PartitionDimension=2  PartitionWidth=1  PartitionOffset=0
  Cast To Double : DataTypeConversion  OutDataTypeStr=double  SaturateOnIntegerOverflow=off  RndMeth=Floor
  Cast To Single : DataTypeConversion  OutDataTypeStr=single  SaturateOnIntegerOverflow=off  RndMeth=Floor
  Constant : Constant  Value=0  OutDataTypeStr=single
  Demux : Demux  Outputs=3
  Direction Cosine Matrix Body to Wind : aerolibtransform2/Direction Cosine Matrix Body to Wind
  Display : Display
  Display1 : Display
  For Each : ForEach  DisableCoverage=on  SpecifiedNumIters=7
  Matrix Multiply : Product  Multiplication=Matrix(*)
  Mux : Mux  Inputs=3
  Mux1 : Mux  Inputs=2
  Transpose : Math  Operator=transpose
  Unary Minus : UnaryMinus
  Unary Minus1 : UnaryMinus
  Fb : Outport  ConcatenationDimension=2
  wires:
  Fw/1 -> Display1/1, Demux/1
  alpha/1 -> Display/1, Mux1/1
  Matrix Multiply/1 -> Fb/1
  Mux/1 -> Matrix Multiply/2
  Demux/1 -> Unary Minus/1
  Unary Minus/1 -> Mux/1
  Demux/2 -> Mux/2
  Unary Minus1/1 -> Mux/3
  Demux/3 -> Unary Minus1/1
  Direction Cosine Matrix Body to Wind/1 -> Transpose/1
  Transpose/1 -> Cast To Single/1
  Mux1/1 -> Cast To Double/1
  Constant/1 -> Mux1/2
  Cast To Single/1 -> Matrix Multiply/1
  Cast To Double/1 -> Direction Cosine Matrix Body to Wind/1

== system unifier_obm/OBM/Aero/WingForces/Right/WingRootForces/WingRootPreLookup ==
  flap_defl : Inport
  alpha : Inport  Port=2
  V_node : Inport  Port=3
  DEP_J : Inport  Port=4
  Constant8 : Constant  Value=0:4
  Prelookup : PreLookup  BreakpointsData=dp_WING_root.flap_defl  IndexSearchMethod=Linear search  BeginIndexSearchUsingPreviousIndexResult=on  UseLastBreakpoint=on
  Prelookup1 : PreLookup  BreakpointsData=dp_WING_root.alphas  IndexSearchMethod=Linear search  BeginIndexSearchUsingPreviousIndexResult=on  UseLastBreakpoint=on
  Prelookup2 : PreLookup  BreakpointsData=dp_WING_root.V  IndexSearchMethod=Linear search  BeginIndexSearchUsingPreviousIndexResult=on  UseLastBreakpoint=on
  Prelookup3 : PreLookup  BreakpointsData=dp_WING_root.DEP_J  IndexSearchMethod=Linear search  BeginIndexSearchUsingPreviousIndexResult=on  UseLastBreakpoint=on
  Out1 : Outport
  Out2 : Outport  Port=2
  Out3 : Outport  Port=3
  Out4 : Outport  Port=4
  Out6 : Outport  Port=5
  Out7 : Outport  Port=6
  Out8 : Outport  Port=7
  Out9 : Outport  Port=8
  Out5 : Outport  Port=9
  wires:
  Prelookup/1 -> Out1/1
  Constant8/1 -> Out5/1
  Prelookup1/2 -> Out4/1
  Prelookup/2 -> Out2/1
  alpha/1 -> Prelookup1/1
  Prelookup1/1 -> Out3/1
  flap_defl/1 -> Prelookup/1
  V_node/1 -> Prelookup2/1
  DEP_J/1 -> Prelookup3/1
  Prelookup2/1 -> Out6/1
  Prelookup2/2 -> Out7/1
  Prelookup3/1 -> Out8/1
  Prelookup3/2 -> Out9/1

== system unifier_obm/OBM/Aero/WingForces/Right/WingTipForces/WingRootPreLookup ==
  ail_defl : Inport
  alpha : Inport  Port=2
  V_node : Inport  Port=3
  DEP_J : Inport  Port=4
  Constant8 : Constant  Value=0:1
  Prelookup : PreLookup  BreakpointsData=dp_WING_tip.ail_defl  IndexSearchMethod=Linear search  BeginIndexSearchUsingPreviousIndexResult=on  UseLastBreakpoint=on
  Prelookup1 : PreLookup  BreakpointsData=dp_WING_tip.alphas  IndexSearchMethod=Linear search  BeginIndexSearchUsingPreviousIndexResult=on  UseLastBreakpoint=on
  Prelookup2 : PreLookup  BreakpointsData=dp_WING_tip.V  IndexSearchMethod=Linear search  BeginIndexSearchUsingPreviousIndexResult=on  UseLastBreakpoint=on
  Prelookup3 : PreLookup  BreakpointsData=dp_WING_tip.DEP_J  IndexSearchMethod=Linear search  BeginIndexSearchUsingPreviousIndexResult=on  UseLastBreakpoint=on
  Out1 : Outport
  Out2 : Outport  Port=2
  Out3 : Outport  Port=3
  Out4 : Outport  Port=4
  Out6 : Outport  Port=5
  Out7 : Outport  Port=6
  Out8 : Outport  Port=7
  Out9 : Outport  Port=8
  Out5 : Outport  Port=9
  wires:
  Prelookup/1 -> Out1/1
  Constant8/1 -> Out5/1
  Prelookup1/2 -> Out4/1
  Prelookup/2 -> Out2/1
  alpha/1 -> Prelookup1/1
  Prelookup1/1 -> Out3/1
  ail_defl/1 -> Prelookup/1
  V_node/1 -> Prelookup2/1
  DEP_J/1 -> Prelookup3/1
  Prelookup2/1 -> Out6/1
  Prelookup2/2 -> Out7/1
  Prelookup3/1 -> Out8/1
  Prelookup3/2 -> Out9/1
